simulink model "Quadrature_Phase_Shift_Keying"  (R2024a)
settings: Solver=VariableStepAuto  StartTime=0.0  StopTime=10.0  RelTol=1e-3
libraries: commdigbbndpm3 x2, commchan3 x1, commrandsrc3 x1
settings Model: Creator=online  LastModifiedBy=online
settings RTWCC: GPUComputeCapability=3.5

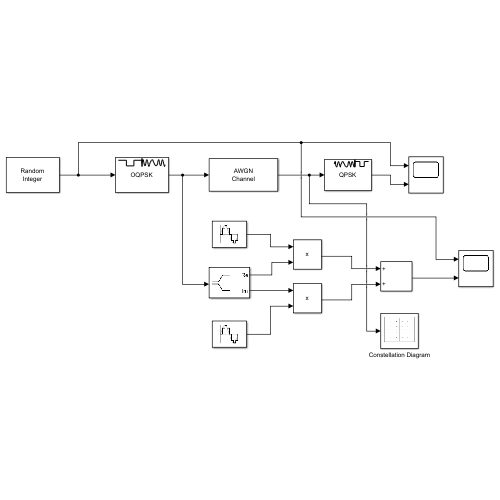
[thumbnail: Simulink's stored preview of the top-level diagram]
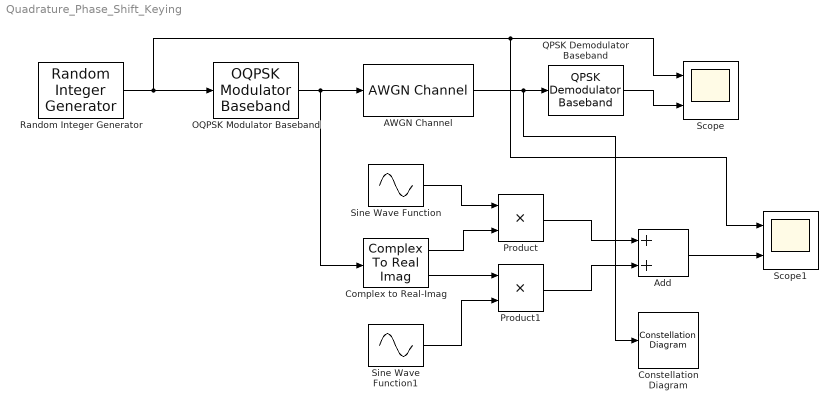
== system Quadrature_Phase_Shift_Keying ==
  AWGN Channel : commchan3/AWGN Channel  LegacyMode=off  NoiseMethod="Signal to noise ratio  (SNR)"  noiseMode="Signal to noise ratio  (SNR)"  EbNo=10  EsNo=10  SNR=10  BitsPerSymbol=1  SignalPower=1  SamplesPerSymbol=1  SymbolPeriod=1  VarianceSource=Parameter  Variance=1  RandomStream=Global stream  Seed=67  SimulateUsing=Code generation
  Add : Sum
  Complex to Real-Imag : ComplexToRealImag
  Constellation Diagram : ConstellationDiagram  WindowPosition=[0.000000,32.000000,1280.000000,657.000000,]  ScopeFrameLocation=window  SymbolsToDisplaySource=Property  SymbolsToDisplay=1000  XLimits=[-2.98,2.98]  YLimits=[-1.38,1.38]
  OQPSK Modulator Baseband : commdigbbndpm3/OQPSK Modulator Baseband  VariantControl=strcmp(pulseShape, 'Custom') && isequal(denom, 1)  InType=Integer  Mapping=Gray  Ph=pi/4  pulseShape=Half sine  num=[0.7071, 0.7071]  denom=[1]  rolloff=0.2  filterSpan=10  sps=4  RateOptions=Enforce single-rate processing  outDtype=double  isIIR=off
  Product : Product
  Product1 : Product
  QPSK Demodulator Baseband : commdigbbndpm3/QPSK Demodulator Baseband  OutType=Integer  DecType=Hard decision  VarSource=Dialog  Variance=1  Dec=Gray  Ph=pi/4  outDtype1=Inherit via internal rule  outDtype2=Inherit via internal rule  derotateFactorWordLen=16  derotateFactorDataTypeStr=Inherit: Same word length as input  derotateFactorLastDataTypeStr=Inherit: Same word length as input
  Random Integer Generator : commrandsrc3/Random Integer Generator  SetSize=4  SeedSource=Auto  Seed=0  SampleTime=1  SamplesPerFrame=1  OutputDataType=double  SimulateUsing=Interpreted execution
  Scope : Scope  NumInputPorts=2
  Scope1 : Scope  NumInputPorts=2
  Sine Wave Function : Sin  Frequency=8*pi  SampleTime=0.001
  Sine Wave Function1 : Sin  Frequency=8*pi  Phase=pi/2  SampleTime=0.001
  wires:
  OQPSK Modulator Baseband/1 -> Complex to Real-Imag/1, AWGN Channel/1
  AWGN Channel/1 -> Constellation Diagram/1, QPSK Demodulator Baseband/1
  QPSK Demodulator Baseband/1 -> Scope/2
  Random Integer Generator/1 -> Scope1/1, Scope/1, OQPSK Modulator Baseband/1
  Product/1 -> Add/1
  Product1/1 -> Add/2
  Complex to Real-Imag/1 -> Product/2
  Complex to Real-Imag/2 -> Product1/1
  Sine Wave Function/1 -> Product/1
  Sine Wave Function1/1 -> Product1/2
  Add/1 -> Scope1/2
